simulink model "lookupTableDynamic_TestGen18"  (R2017b)
settings: Solver=FixedStepDiscrete  StartTime=0.0  StopTime=10.0  RelTol=1e-3
libraries: simulink x1
settings Model: Creator=ktrinh  LastModifiedBy=ktrinh
settings DebuggingCC: ParameterOverflowMsg=none

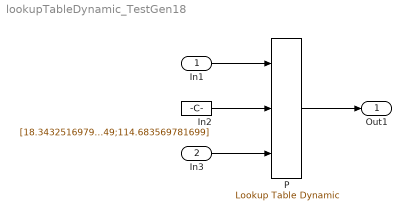
== system lookupTableDynamic_TestGen18 ==
  In1 : Inport  OutMin=16.3433  OutMax=116.6836  OutDataTypeStr=single  PortDimensions=3
  In3 : Inport  Port=2  PortDimensions=5
  In2 : Constant  Value=[18.3432516979302;29.7023915410528;80.9065496324858;99.7198032665349;114.683569781699]  OutDataTypeStr=single
  P : simulink/Lookup Tables/Lookup Table Dynamic  LookUpMeth=Use Input Nearest  OutDataType=fixdt('double')  OutScaling=2^-10  OutDataTypeStr=Inherit: Inherit via back propagation  RndMeth=Round  DoSatur=off
      settings: SourceProductName=Simulink
  Out1 : Outport
  wires:
  In1/1 -> P/1
  In2/1 -> P/2
  In3/1 -> P/3
  P/1 -> Out1/1
